simulink model "SP_Simulink"  (R2021b)
settings: Solver=VariableStepAuto  StartTime=0.0  StopTime=10.0  RelTol=1e-3
values from neighbouring files (symbols this model uses):
  g = 9.80665    [SP_Parameters.m]
  k = 0.2    [SP_Parameters.m]
  l = 1.5    [SP_Parameters.m]
  S0 = [pi/4 ,2]    [SP_Parameters.m]
settings Model: Creator=Sushmanth Sai G  LastModifiedBy=Sushmanth Sai G

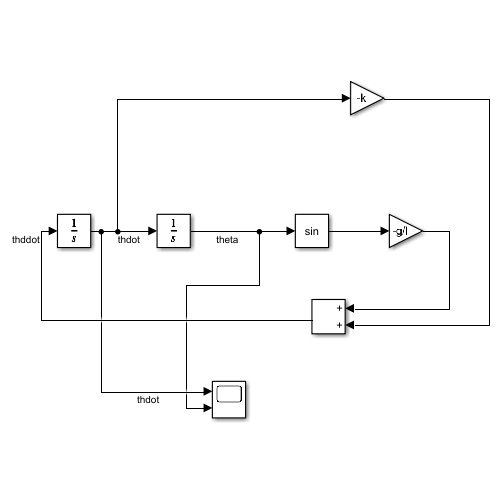
[thumbnail: Simulink's stored preview of the top-level diagram]
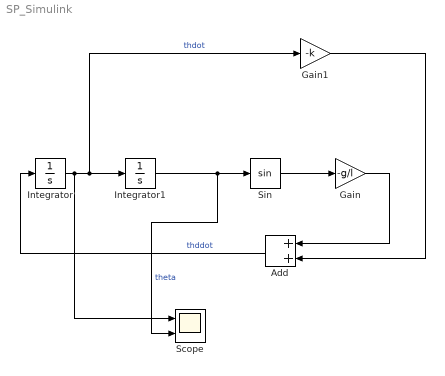
== system SP_Simulink ==
  Add : Sum
  Gain : Gain  Gain=-g/l
  Gain1 : Gain  Gain=-k
  Integrator : Integrator  InitialCondition=S0(2)
  Integrator1 : Integrator  InitialCondition=S0(1)
  Scope : Scope  NumInputPorts=2
  Sin : Trigonometry
  wires:
  Integrator/1 -> Scope/1, Gain1/1, Integrator1/1  "thdot"
  Add/1 -> Integrator/1  "thddot"
  Integrator1/1 -> Scope/2, Sin/1  "theta"
  Sin/1 -> Gain/1
  Gain/1 -> Add/1
  Gain1/1 -> Add/2
